simulink model "Model"  (R2021a)
settings: Solver=VariableStepAuto  StartTime=0.0  StopTime=1  RelTol=1e-3
PreLoadFcn:
  | Pmin = 50e3*.15;
  | V = 380;
  | f = 60;
  | fsw = 5e3;
  | Lf = ((.1*V^2)/(2*pi*f*Pmin));
  | RLf = Lf*25;
undefined symbols (not defined in the file or in its folder): sigbuilder_block
libraries: spsThreePhaseSeriesRLCLoadLib x11, spsThreePhaseVIMeasurementLib x4, spsThreePhaseHarmonicFilterLib x3, spsIdealSwitchLib x3, pid_lib x2, spsThreePhaseBreakerLib x1, spsImpedanceMeasurementLib x1, spsPWMGenerator2LevelLib x1, spsThreePhaseSeriesRLCBranchLib x1, spsUniversalBridgeLib x1, spsabctodq0Lib x1, spsdq0toabcLib x1
settings Model: Creator=SHANTO  LastModifiedBy=SHANTO

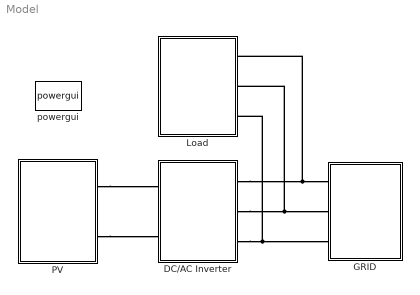
== system Model ==
  DC/AC Inverter : Subsystem
      mask Display: image('$imagefile'); % Use "Edit Image" on toolstrip to change.
  GRID : Subsystem
      mask Display: image('$imagefile'); % Use "Edit Image" on toolstrip to change.
  Load : Subsystem
      mask Display: image('$imagefile'); % Use "Edit Image" on toolstrip to change.
  "PV " : Subsystem
      mask Display: image('$imagefile'); % Use "Edit Image" on toolstrip to change.
  powergui : spspowerguiLib/powergui  Priority=1  SimulationMode=Discrete  SampleTime=1e-06  frequency=60  Iterations=50  frequencyindice=0  Pbase=100e6  ErrMax=1e-4  UnitsV=kV  UnitsW=MW  buscounter=0  FunctionMessages=off  echomessages=off  EnableUseOfTLC=off  CurrentSourceSwitches=off  DisableSnubberDevices=off  DisableRonSwitches=off  DisableVfSwitches=off  DisplayEquations=off  AutomaticDiscreteSolvers=off  SolverType=Tustin/Backward Euler (TBE)  Interpol=off  ExternalGateDelay=off  methode=off  Ts=100  x0status=blocks  SPID=on  SwTol=0  HookPort=off  NonlinearTolerance=1e-4  nMaxIteration=100  ContinueOnMaxIteration=off  RestoreLinks=warning  ResistiveCurrentMeasurement=off  Frange=[0:2:500]  Ylog=off  Xlog=on  ShowGrid=off  save=off  variable=ZData  structure=0  ZoomFFT=off  StartTime=0.0  cycles=1  DisplayStyle=1  fundamental=60  FreqAxis=off  MaxFrequency=1000  frequencyindicesteady=1  RmsSteady=1  display=off
  connections:
  "PV "/RConn1 -- DC/AC Inverter/LConn1
  "PV "/RConn2 -- DC/AC Inverter/LConn2
  DC/AC Inverter/RConn1 -- Load/RConn1 -- GRID/LConn1
  DC/AC Inverter/RConn2 -- GRID/LConn2 -- Load/RConn2
  DC/AC Inverter/RConn3 -- GRID/LConn3 -- Load/RConn3

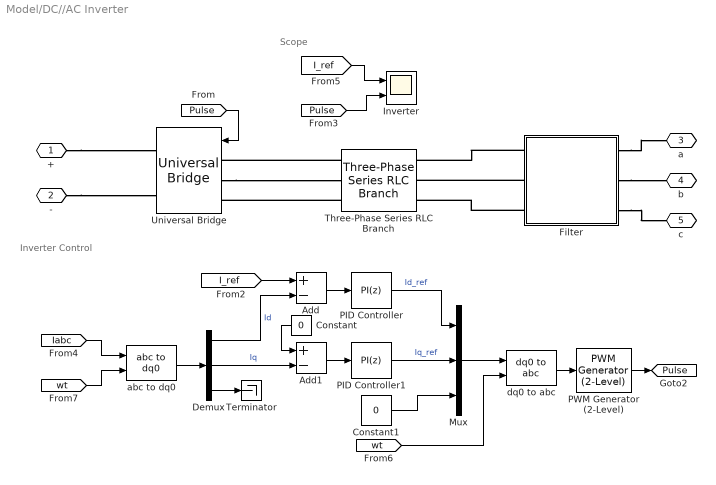
== system Model/DC//AC Inverter ==
  note: Scope
  note: Inverter Control
  Add : Sum  Inputs=+-
  Add1 : Sum  Inputs=+-
  Constant : Constant  Value=0
  Constant1 : Constant  Value=0
  Demux : Demux  Outputs=3
  Filter : Subsystem
  Inverter : Scope  NumInputPorts=2
  Mux : Mux  Inputs=3
  PID Controller : pid_lib/PID Controller  Controller=PI  Form=Parallel  TimeDomain=Discrete-time  UseExternalTs=off  SampleTime=1e-06  IntegratorMethod=Forward Euler  FilterMethod=Forward Euler  ControllerParametersSource=internal  P=0.005  I=1  D=0  UseFilter=on  N=100  TunerSelectOption=Transfer Function Based (PID Tuner App)  InitialConditionSource=internal  InitialConditionForIntegrator=0  InitialConditionForFilter=0  DifferentiatorICPrevScaledInput=0  ExternalReset=none  TrackingMode=off  Kt=1  LimitOutput=on  SatLimitsSource=internal  UpperSaturationLimit=1.2  LowerSaturationLimit=0  LinearizeAsGain=on  AntiWindupMode=none  Kb=1  POutMin=[]  POutMax=[]  IOutMin=[]  IOutMax=[]  DOutMin=[]  DOutMax=[]  NOutMin=[]  NOutMax=[]  SumOutMin=[]  SumOutMax=[]  SaturationOutMin=[]  SaturationOutMax=[]  PParamMin=[]  PParamMax=[]  IParamMin=[]  IParamMax=[]  DParamMin=[]  DParamMax=[]  NParamMin=[]  NParamMax=[]  KbParamMin=[]  KbParamMax=[]  KtParamMin=[]  KtParamMax=[]  KbOutMin=[]  KbOutMax=[]  KtOutMin=[]  KtOutMax=[]  IntegratorOutMin=[]  IntegratorOutMax=[]  FilterOutMin=[]  FilterOutMax=[]  SumI1OutMin=[]  SumI1OutMax=[]  SumI2OutMin=[]  SumI2OutMax=[]  SumI3OutMin=[]  SumI3OutMax=[]  SumI4OutMin=[]  SumI4OutMax=[]  SumDOutMin=[]  SumDOutMax=[]  DifferentiatorOutMin=[]  DifferentiatorOutMax=[]  FilterDiffOutCoefMin=[]  FilterDiffOutCoefMax=[]  ReciprocalOutMin=[]  ReciprocalOutMax=[]  SumDenOutMin=[]  SumDenOutMax=[]  SumNumOutMin=[]  SumNumOutMax=[]  DivideOutMin=[]  DivideOutMax=[]  UdiffTsProdOutMin=[]  UdiffTsProdOutMax=[]  NTsProdOutMin=[]  NTsProdOutMax=[]  UintegralTsProdOutMin=[]  UintegralTsProdOutMax=[]  UngainTsProdOutMin=[]  UngainTsProdOutMax=[]  IntegratorContinuousStateAttributes=''  IntegratorStateMustResolveToSignalObject=off  IntegratorRTWStateStorageClass=Auto  FilterContinuousStateAttributes=''  FilterStateMustResolveToSignalObject=off  FilterRTWStateStorageClass=Auto  ParallelPVariant=InternalParameters  IdealPVariant=Disabled  IVariant=InternalParameters  DVariant=Disabled  IntegratorVariant=Discrete  SatVariant=Enabled  AWVariant=Passthrough  PCopyVariant=Disabled  TRVariant=Disabled  FdbkBlocksVariant=Forward  IdealPFdbkVariant=Disabled  SatFdbkVariant=Disabled  DerivativeFilterVariant=Disabled  NVariant=Disabled  NCopyVariant=Disabled_SignalSpec  FilterICVariant=Disabled  IntegratorICVariant=InternalICs  ExternalResetVariant=Disabled  TRSumVariant=Passthrough  SumFdbkVariant=Disabled  SumVariant=Sum_PI  TsampFilterVariant=InternalTs  TsampNgainVariant=Passthrough  TsampIntegralVariant=Passthrough  ExternalSaturationOutDataTypeStr=Inherit: Same as second input
  PID Controller1 : pid_lib/PID Controller  Controller=PI  Form=Parallel  TimeDomain=Discrete-time  UseExternalTs=off  SampleTime=1e-05  IntegratorMethod=Forward Euler  FilterMethod=Forward Euler  ControllerParametersSource=internal  P=0.005  I=1  D=0  UseFilter=on  N=100  TunerSelectOption=Transfer Function Based (PID Tuner App)  InitialConditionSource=internal  InitialConditionForIntegrator=0  InitialConditionForFilter=0  DifferentiatorICPrevScaledInput=0  ExternalReset=none  TrackingMode=off  Kt=1  LimitOutput=on  SatLimitsSource=internal  UpperSaturationLimit=1.2  LowerSaturationLimit=0  LinearizeAsGain=on  AntiWindupMode=none  Kb=1  POutMin=[]  POutMax=[]  IOutMin=[]  IOutMax=[]  DOutMin=[]  DOutMax=[]  NOutMin=[]  NOutMax=[]  SumOutMin=[]  SumOutMax=[]  SaturationOutMin=[]  SaturationOutMax=[]  PParamMin=[]  PParamMax=[]  IParamMin=[]  IParamMax=[]  DParamMin=[]  DParamMax=[]  NParamMin=[]  NParamMax=[]  KbParamMin=[]  KbParamMax=[]  KtParamMin=[]  KtParamMax=[]  KbOutMin=[]  KbOutMax=[]  KtOutMin=[]  KtOutMax=[]  IntegratorOutMin=[]  IntegratorOutMax=[]  FilterOutMin=[]  FilterOutMax=[]  SumI1OutMin=[]  SumI1OutMax=[]  SumI2OutMin=[]  SumI2OutMax=[]  SumI3OutMin=[]  SumI3OutMax=[]  SumI4OutMin=[]  SumI4OutMax=[]  SumDOutMin=[]  SumDOutMax=[]  DifferentiatorOutMin=[]  DifferentiatorOutMax=[]  FilterDiffOutCoefMin=[]  FilterDiffOutCoefMax=[]  ReciprocalOutMin=[]  ReciprocalOutMax=[]  SumDenOutMin=[]  SumDenOutMax=[]  SumNumOutMin=[]  SumNumOutMax=[]  DivideOutMin=[]  DivideOutMax=[]  UdiffTsProdOutMin=[]  UdiffTsProdOutMax=[]  NTsProdOutMin=[]  NTsProdOutMax=[]  UintegralTsProdOutMin=[]  UintegralTsProdOutMax=[]  UngainTsProdOutMin=[]  UngainTsProdOutMax=[]  IntegratorContinuousStateAttributes=''  IntegratorStateMustResolveToSignalObject=off  IntegratorRTWStateStorageClass=Auto  FilterContinuousStateAttributes=''  FilterStateMustResolveToSignalObject=off  FilterRTWStateStorageClass=Auto  ParallelPVariant=InternalParameters  IdealPVariant=Disabled  IVariant=InternalParameters  DVariant=Disabled  IntegratorVariant=Discrete  SatVariant=Enabled  AWVariant=Passthrough  PCopyVariant=Disabled  TRVariant=Disabled  FdbkBlocksVariant=Forward  IdealPFdbkVariant=Disabled  SatFdbkVariant=Disabled  DerivativeFilterVariant=Disabled  NVariant=Disabled  NCopyVariant=Disabled_SignalSpec  FilterICVariant=Disabled  IntegratorICVariant=InternalICs  ExternalResetVariant=Disabled  TRSumVariant=Passthrough  SumFdbkVariant=Disabled  SumVariant=Sum_PI  TsampFilterVariant=InternalTs  TsampNgainVariant=Passthrough  TsampIntegralVariant=Passthrough  ExternalSaturationOutDataTypeStr=Inherit: Same as second input
  PWM Generator (2-Level) : spsPWMGenerator2LevelLib/PWM Generator (2-Level)  ModulatorType=Three-phase bridge (6 pulses)  ModulatorMode=Unsynchronized  Fc=fsw  Pc=90  nF=27  MinMax="[ -1  1 ]"  SamplingTechnique=Natural  ModulatingSignals=off  m=0.8  Freq=60  Phase=0  Ts=1e-6  ShowCarrierOutport=off
  Terminator : Terminator
  Three-Phase Series RLC Branch : spsThreePhaseSeriesRLCBranchLib/Three-Phase Series RLC Branch  LConnTagsString=A|B|C  RConnTagsString=A|B|C  BranchType=RL  Resistance=RLf  Inductance=Lf  Capacitance=1e-6  Measurements=None
  Universal Bridge : spsUniversalBridgeLib/Universal Bridge  Arms=3  SnubberResistance=1e5  SnubberCapacitance=inf  Device=IGBT / Diodes  Ron=1e-3  Lon=0  ForwardVoltages="[  0  0  ]"  ForwardVoltage=0  GTOparameters=[ 10e-6 , 20e-6 ]  IGBTparameters=[ 1e-6 , 2e-6 ]  Measurements=None  Measurements_2=None  converterType=Rectifier
  abc to dq0 : spsabctodq0Lib/abc to dq0  Alignment=90 degrees behind phase A axis
  dq0 to abc : spsdq0toabcLib/dq0 to abc  Alignment=90 degrees behind phase A axis
  + : PMIOPort  Side=Left
  - : PMIOPort  Port=2  Side=Left
  a : PMIOPort  Port=3  Side=Right
  b : PMIOPort  Port=4  Side=Right
  c : PMIOPort  Port=5  Side=Right
  tag scope: Pulse=global
  wires:
  [wt] -> abc to dq0/2
  Add1/1 -> PID Controller1/1
  Demux/2 -> Add1/2  "Iq"
  PID Controller1/1 -> Mux/2  "Iq_ref"
  PID Controller/1 -> Mux/1  "Id_ref"
  Constant/1 -> Add1/1
  Demux/1 -> Add/2  "Id"
  Add/1 -> PID Controller/1
  dq0 to abc/1 -> PWM Generator (2-Level)/1
  Mux/1 -> dq0 to abc/1
  Constant1/1 -> Mux/3
  abc to dq0/1 -> Demux/1
  [wt] -> dq0 to abc/2
  [Iabc] -> abc to dq0/1
  PWM Generator (2-Level)/1 -> [Pulse]
  Demux/3 -> Terminator/1
  [Pulse] -> Universal Bridge/1
  [I_ref] -> Add/1
  [I_ref] -> Inverter/1
  [Pulse] -> Inverter/2
  connections:
  Universal Bridge/LConn2 -- Three-Phase Series RLC Branch/LConn2
  Three-Phase Series RLC Branch/LConn3 -- Universal Bridge/LConn3
  -/RConn1 -- Universal Bridge/RConn2
  Filter/RConn2 -- Three-Phase Series RLC Branch/RConn2
  +/RConn1 -- Universal Bridge/RConn1
  Filter/RConn3 -- Three-Phase Series RLC Branch/RConn3
  Three-Phase Series RLC Branch/LConn1 -- Universal Bridge/LConn1
  Filter/RConn1 -- Three-Phase Series RLC Branch/RConn1
  Filter/LConn2 -- b/RConn1
  Filter/LConn1 -- a/RConn1
  Filter/LConn3 -- c/RConn1

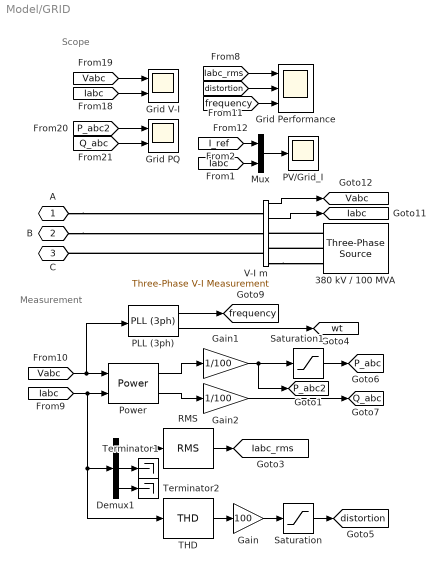
== system Model/GRID ==
  note: Scope
  note: Measurement
  380 kV / 100 MVA : spsThreePhaseSourceLib/Three-Phase Source  InternalConnection=Yg  VoltagePhases=off  Voltage=380  PhaseAngle=0  Voltage_phases=[25e3 25e3 25e3]/sqrt(3)  PhaseAngles_phases=[0 -120 +120]  Frequency=60  NonIdealSource=on  SpecifyImpedance=on  Resistance=1e-4  Inductance=0.2e-6  ShortCircuitLevel=100e6  BaseVoltage=380  XRratio=7  BusType=PQ  Pref=2.5e6  Qref=0  Prefabc=[10e3, 10e3, 10e3]  Qrefabc=[0, 0, 0]  Qmin=-inf  Qmax=inf
  Demux1 : Demux  Outputs=3
  Gain : Gain  Gain=100
  Gain1 : Gain  Gain=1/100
  Gain2 : Gain  Gain=1/100
  Grid PQ : Scope  NumInputPorts=2
  Grid Performance : Scope  NumInputPorts=3
  Grid V-I : Scope  NumInputPorts=2
  Mux : Mux  Inputs=2
  PLL (3ph) : spsPLL3phLib/PLL (3ph)  Fmin=45  Par_Init=[0, 60]  ParK=[180, 3200, 1]  TcD=1e-4  MaxRateChangeFreq=12  FilterCutOffFreq=25  Ts=1e-6  AGC=on
  PV/Grid_I : Scope
  Power : spsPowerLib/Power  Freq=60  Vinit=[1, 0]  Iinit=[1, 0]  Ts=0
      settings: SourceProductBaseCode=PS
  RMS : spsRMSLib/RMS  TrueRMS=on  Freq=60  RMSInit=120  Ts=1e-6
  Saturation : Saturate  UpperLimit=50  LowerLimit=0
  Saturation1 : Saturate  UpperLimit=60  LowerLimit=0
  THD : spsTHDLib/THD  Freq=60  Ts=1e-6
      settings: SourceProductBaseCode=PS
  Terminator1 : Terminator
  Terminator2 : Terminator
  V-I m : spsThreePhaseVIMeasurementLib/Three-Phase V-I Measurement  VoltageMeasurement=phase-to-ground  SetLabelV=off  LabelV=PV_Vabc  Vpu=off  VpuLL=off  CurrentMeasurement=yes  SetLabelI=off  LabelI=PV_Iabc  Ipu=off  Pbase=100e6  Vbase=500e3  OutputType=Complex  PhasorSimulation=off  PSBequivalent=0
  A : PMIOPort  Side=Left
  B : PMIOPort  Port=2  Side=Left
  C : PMIOPort  Port=3  Side=Left
  tag scope: Iabc=global, Iabc_rms=global, P_abc2=global, P_abc=global, Q_abc=global, Vabc=global, distortion=global, frequency=global, wt=global
  wires:
  V-I m/2 -> [Iabc]
  V-I m/1 -> [Vabc]
  [frequency] -> Grid Performance/3
  PLL (3ph)/2 -> [wt]
  PLL (3ph)/1 -> [frequency]
  [distortion] -> Grid Performance/2
  Power/2 -> Gain2/1
  Gain2/1 -> [Q_abc]
  [Iabc_rms] -> Grid Performance/1
  Demux1/1 -> RMS/1
  Power/1 -> Gain1/1
  THD/1 -> Gain/1
  Demux1/2 -> Terminator1/1
  [Iabc] -> Power/2, THD/1, Demux1/1
  [Vabc] -> PLL (3ph)/1, Power/1
  Demux1/3 -> Terminator2/1
  Saturation1/1 -> [P_abc]
  Gain/1 -> Saturation/1
  Gain1/1 -> [P_abc2], Saturation1/1
  Saturation/1 -> [distortion]
  RMS/1 -> [Iabc_rms]
  [Vabc] -> Grid V-I/1
  [Iabc] -> Grid V-I/2
  [Q_abc] -> Grid PQ/2
  [P_abc2] -> Grid PQ/1
  Mux/1 -> PV/Grid_I/1
  [Iabc] -> Mux/2
  [I_ref] -> Mux/1
  connections:
  380 kV / 100 MVA/RConn1 -- V-I m/RConn1
  V-I m/RConn3 -- 380 kV / 100 MVA/RConn3
  380 kV / 100 MVA/RConn2 -- V-I m/RConn2
  A/RConn1 -- V-I m/LConn1
  B/RConn1 -- V-I m/LConn2
  V-I m/LConn3 -- C/RConn1

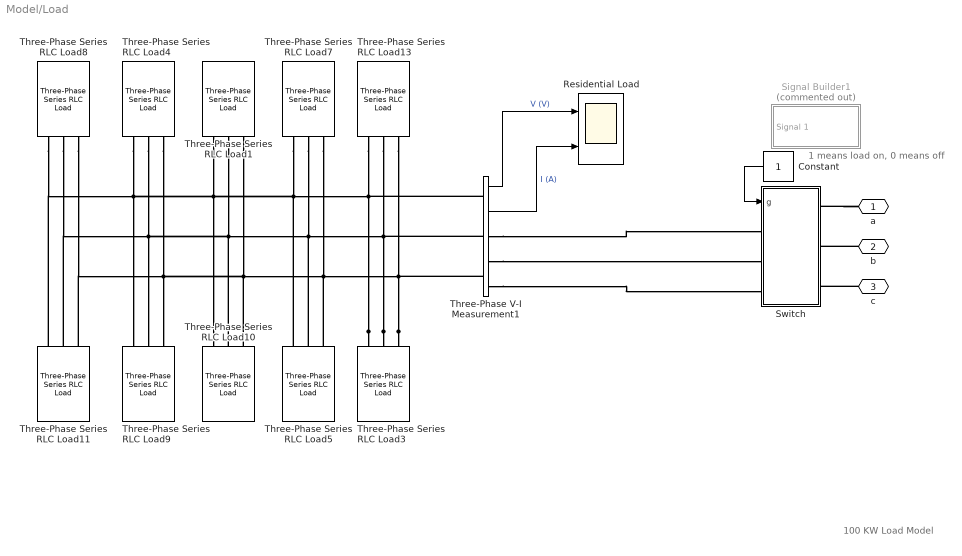
== system Model/Load ==
  note: 1 means load on, 0 means off
  note: 100 KW Load Model
  Constant : Constant
  Residential Load : Scope  NumInputPorts=2
  Signal Builder1 : Subsystem  Tag=STV Subsys  Commented=on  LoadFcn=sigbuilder_block('load');  StartFcn=sigbuilder_block('start');  StopFcn=sigbuilder_block('stop');  ClipboardFcn=sigbuilder_block('clipboard');  mask(Sigbuilder block){tuvar=[0:10]}
      mask help: Simulink:masks:SigbuilderBlock_MD
      mask init:
      | if ~strcmp(get_param(bdroot(gcbh),'SimulationStatus'),'stopped') tuvar = sigbuilder_block('maskInit'); end
      settings: CopyFcn=sigbuilder_block('copy');  DeleteFcn=sigbuilder_block('delete');  ModelCloseFcn=sigbuilder_block('modelClose');  PreSaveFcn=sigbuilder_block('preSave');  PauseFcn=sigbuilder_block('pause');  ContinueFcn=sigbuilder_block('continue');  NameChangeFcn=sigbuilder_block('namechange');  OpenFcn=sigbuilder_block('open',[437.6 199.2 550.4 400 ]);  CloseFcn=sigbuilder_block('close');
      mask Display: plot(0, 0, 100, 100,[2, 2, 32, 32, 2], [68, 8, 8, 68, 68],[32, 2], [38, 38], [32, 19, 2],[53, 60, 44], [32, 17, 17, 2],[16, 16, 31, 31]);txt = getActiveGroup(gcbh);text(2, 100, txt,'verticalAlignment', 'top');
  Switch : Subsystem
  Three-Phase Series RLC Load{1,3..5,7..11,13} (10 alike) : spsThreePhaseSeriesRLCLoadLib/Three-Phase Series RLC Load  LConnTagsString=A|B|C  Configuration=Y (grounded)  NominalVoltage=380  Vabc=[1e3 1e3 1e3]  Vabcp=[1e3 1e3 1e3]  NominalFrequency=60  UnbalancedPower=off  ActivePower=10e3  InductivePower=100  CapacitivePower=100  Pabc=[10e3 9e3 11e3]  QLabc=[100 90 110]  QCabc=[100 90 110]  Pabcp=[10e3 9e3 11e3]  QLabcp=[100 90 110]  QCabcp=[100 90 110]  Measurements=None  LoadType=constant Z
  Three-Phase V-I Measurement1 : spsThreePhaseVIMeasurementLib/Three-Phase V-I Measurement  VoltageMeasurement=phase-to-ground  SetLabelV=off  LabelV=Vabc_load2  Vpu=off  VpuLL=off  CurrentMeasurement=yes  SetLabelI=off  LabelI=Iabc_load2  Ipu=off  Pbase=100e6  Vbase=500e3  OutputType=Complex  PhasorSimulation=off  PSBequivalent=0
  a : PMIOPort  Side=Right
  b : PMIOPort  Port=2  Side=Right
  c : PMIOPort  Port=3  Side=Right
  wires:
  Three-Phase V-I Measurement1/2 -> Residential Load/2  "I (A)"
  Three-Phase V-I Measurement1/1 -> Residential Load/1  "V (V)"
  Constant/1 -> Switch/1(g)
  connections:
  Three-Phase V-I Measurement1/RConn3 -- Switch/LConn3
  Three-Phase Series RLC Load3/LConn1 -- Three-Phase V-I Measurement1/LConn1 -- Three-Phase Series RLC Load13/LConn1 -- Three-Phase Series RLC Load8/LConn1 -- Three-Phase Series RLC Load11/LConn1 -- Three-Phase Series RLC Load4/LConn1 -- Three-Phase Series RLC Load9/LConn1 -- Three-Phase Series RLC Load1/LConn1 -- Three-Phase Series RLC Load10/LConn1 -- Three-Phase Series RLC Load7/LConn1 -- Three-Phase Series RLC Load5/LConn1
  Three-Phase V-I Measurement1/RConn2 -- Switch/LConn2
  Three-Phase Series RLC Load3/LConn3 -- Three-Phase Series RLC Load10/LConn3 -- Three-Phase Series RLC Load8/LConn3 -- Three-Phase Series RLC Load11/LConn3 -- Three-Phase Series RLC Load4/LConn3 -- Three-Phase Series RLC Load9/LConn3 -- Three-Phase Series RLC Load1/LConn3 -- Three-Phase Series RLC Load7/LConn3 -- Three-Phase Series RLC Load5/LConn3 -- Three-Phase V-I Measurement1/LConn3 -- Three-Phase Series RLC Load13/LConn3
  Three-Phase Series RLC Load3/LConn2 -- Three-Phase V-I Measurement1/LConn2 -- Three-Phase Series RLC Load13/LConn2 -- Three-Phase Series RLC Load8/LConn2 -- Three-Phase Series RLC Load11/LConn2 -- Three-Phase Series RLC Load4/LConn2 -- Three-Phase Series RLC Load9/LConn2 -- Three-Phase Series RLC Load1/LConn2 -- Three-Phase Series RLC Load10/LConn2 -- Three-Phase Series RLC Load7/LConn2 -- Three-Phase Series RLC Load5/LConn2
  Three-Phase V-I Measurement1/RConn1 -- Switch/LConn1
  c/RConn1 -- Switch/RConn3
  b/RConn1 -- Switch/RConn2
  a/RConn1 -- Switch/RConn1

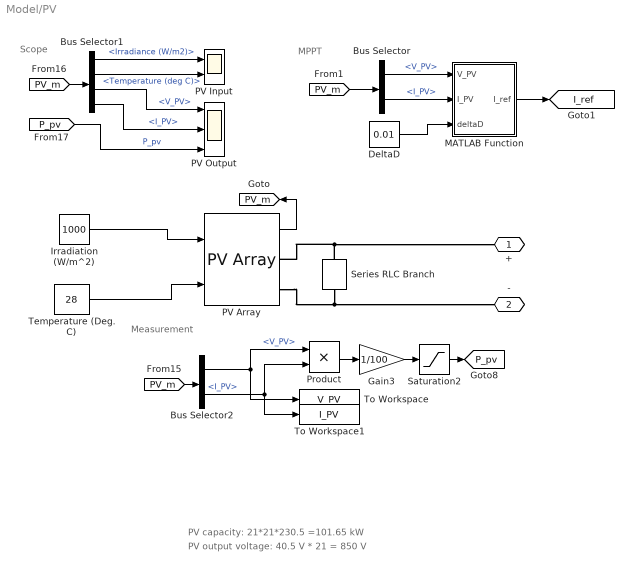
== system Model/PV  ==
  note: PV output voltage: 40.5 V * 21 = 850 V
  note: PV capacity: 21*21*230.5 =101.65 kW
  note: Scope
  note: Measurement
  note: MPPT
  Bus Selector : BusSelector  OutputSignals=V_PV,I_PV
  Bus Selector1 : BusSelector  OutputSignals=Irradiance (W/m2),Temperature (deg C),V_PV,I_PV
  Bus Selector2 : BusSelector  OutputSignals=V_PV,I_PV
  DeltaD : Constant  Value=0.01
  Gain3 : Gain  Gain=1/100
  Irradiation (W/m^2) : Constant  Value=1000
  MATLAB Function : MATLAB Function  TreatAsAtomicUnit=on
  PV Array : spsPVArrayLib/PV Array  Npar=21  Nser=21  PlotType=one module @ 25 deg.C & specified irradiances  S_vec=[1000 600 400 100]  Temp_C_vec="[ 45 25  ]"  ModuleName=SunPower SPR-230E-WHT-D  PlotWhenSelected=off  Pm=230.04  Ncell=72  Voc=48.2  Isc=6.05  Vm=40.5  Im=5.68  beta_Voc_pc=-0.31  alpha_Isc_pc=0.016  beta_Voc=-0.14942  alpha_Isc=0.000968  IL=6.0553  I0=2.9343e-11  nI=1.0009  Rsh=396.8073  Rs=0.34627  RobustModel=off  RobustCellTemperature=313.3991  BAL=on  Tc=1e-6  Tfilter=5e-5
  PV Input : Scope  NumInputPorts=2
  PV Output : Scope  NumInputPorts=3
  Product : Product
  Saturation2 : Saturate  UpperLimit=60  LowerLimit=0
  Series RLC Branch : spsSeriesRLCBranchLib/Series RLC Branch  LConnTagsString=__new0  RConnTagsString=__new0  BranchType=RC  Resistance=1e-3  Inductance=1e-3  SetiL0=off  InitialCurrent=0  Capacitance=100e-6  Setx0=off  InitialVoltage=0  Measurements=None
  Temperature (Deg. C) : Constant  Value=28
  To Workspace : ToWorkspace  VariableName=V_PV  SaveFormat=Timeseries  SampleTime=-1
  To Workspace1 : ToWorkspace  VariableName=I_PV  SaveFormat=Timeseries  SampleTime=-1
  + : PMIOPort  Side=Right
  - : PMIOPort  Port=2  Side=Right
  tag scope: I_ref=global, PV_m=global, P_pv=global
  wires:
  PV Array/1 -> [PV_m]
  [P_pv] -> PV Output/3  "P_pv"
  [PV_m] -> Bus Selector1/1
  Irradiation (W/m^2)/1 -> PV Array/1
  Temperature (Deg. C)/1 -> PV Array/2
  Saturation2/1 -> [P_pv]
  Gain3/1 -> Saturation2/1
  [PV_m] -> Bus Selector2/1
  Bus Selector2/1 -> Product/1, To Workspace/1  "<V_PV>"
  Bus Selector2/2 -> Product/2, To Workspace1/1  "<I_PV>"
  Product/1 -> Gain3/1
  Bus Selector/2 -> MATLAB Function/2(I_PV)  "<I_PV>"
  Bus Selector/1 -> MATLAB Function/1(V_PV)  "<V_PV>"
  [PV_m] -> Bus Selector/1
  DeltaD/1 -> MATLAB Function/3(deltaD)
  MATLAB Function/1(I_ref) -> [I_ref]
  Bus Selector1/1 -> PV Input/1  "<Irradiance (W/m2)>"
  Bus Selector1/2 -> PV Input/2  "<Temperature (deg C)>"
  Bus Selector1/3 -> PV Output/1  "<V_PV>"
  Bus Selector1/4 -> PV Output/2  "<I_PV>"
  connections:
  Series RLC Branch/RConn1 -- PV Array/RConn2 -- -/RConn1
  Series RLC Branch/LConn1 -- +/RConn1 -- PV Array/RConn1

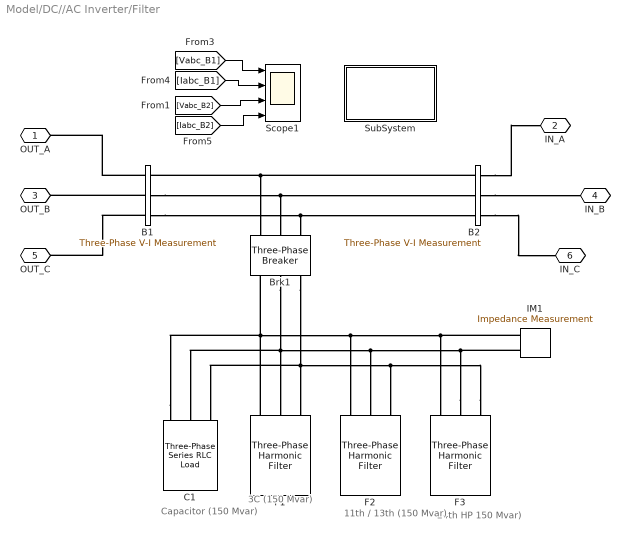
== system Model/DC//AC Inverter/Filter ==
  note: Capacitor
      | (150 Mvar)
  note: 24th HP
      | 150 Mvar)
  note: 11th / 13th
      | (150 Mvar)
  note: 3C
      | (150 Mvar)
  B1 : spsThreePhaseVIMeasurementLib/Three-Phase V-I Measurement  VoltageMeasurement=phase-to-ground  SetLabelV=on  LabelV=Vabc_B1  Vpu=off  VpuLL=off  CurrentMeasurement=yes  SetLabelI=on  LabelI=Iabc_B1  Ipu=off  Pbase=100e6  Vbase=500e3  OutputType=Magnitude  PhasorSimulation=off  PSBequivalent=0
  "B2 " : spsThreePhaseVIMeasurementLib/Three-Phase V-I Measurement  VoltageMeasurement=phase-to-ground  SetLabelV=on  LabelV=Vabc_B2  Vpu=off  VpuLL=off  CurrentMeasurement=yes  SetLabelI=on  LabelI=Iabc_B2  Ipu=off  Pbase=100e6  Vbase=500e3  OutputType=Magnitude  PhasorSimulation=off  PSBequivalent=0
  Brk1 : spsThreePhaseBreakerLib/Three-Phase Breaker  InitialState=closed  SwitchA=off  SwitchB=off  SwitchC=off  SwitchTimes="[4/60  10/60]"  External=off  BreakerResistance=1e-4  SnubberResistance=1e6  SnubberCapacitance=inf  Measurements=None
      settings: AttributesFormatString=\n
  C1 : spsThreePhaseSeriesRLCLoadLib/Three-Phase Series RLC Load  LConnTagsString=A|B|C  Configuration=Y (grounded)  NominalVoltage=500e3  Vabc=[1e3 1e3 1e3]  Vabcp=[1e3 1e3 1e3]  NominalFrequency=60  UnbalancedPower=off  ActivePower=0  InductivePower=0  CapacitivePower=150e6  Pabc=[10e3 9e3 11e3]  QLabc=[100 90 110]  QCabc=[100 90 110]  Pabcp=[10e3 9e3 11e3]  QLabcp=[100 90 110]  QCabcp=[100 90 110]  Measurements=None  LoadType=constant Z
  "F1 " : spsThreePhaseHarmonicFilterLib/Three-Phase Harmonic Filter  LConnTagsString=A|B|C  FilterType=C-type High-pass  FilterConnection=Y (grounded)  ParNom=[500e3 60]  Qc=150e6  Fr=[3*60]  Frd=[11*60 13*60]  Q=2  Measurements=None
      settings: AttributesFormatString=\n  SourceProductBaseCode=PS
  F2 : spsThreePhaseHarmonicFilterLib/Three-Phase Harmonic Filter  LConnTagsString=A|B|C  FilterType=Double-tuned  FilterConnection=Y (grounded)  ParNom=[500e3 60]  Qc=150e6  Fr=[3*60]  Frd=[11*60 13*60]  Q=20  Measurements=None
      settings: AttributesFormatString=\n  SourceProductBaseCode=PS
  F3 : spsThreePhaseHarmonicFilterLib/Three-Phase Harmonic Filter  LConnTagsString=A|B|C  FilterType=High-pass  FilterConnection=Y (grounded)  ParNom=[500e3 60]  Qc=150e6  Fr=[24*60]  Frd=[11*60 13*60]  Q=7  Measurements=None
      settings: AttributesFormatString=\n  SourceProductBaseCode=PS
  IM1 : spsImpedanceMeasurementLib/Impedance Measurement  LConnTagsString=+|-  Factor=0.5
      settings: SourceProductBaseCode=PS
  Scope1 : Scope  NumInputPorts=4
  SubSystem : Subsystem
      settings: OpenFcn=openfig('filters_impedance.fig');
      mask Display: disp('Show\nfilters impedance\nvs\nfrequency')
  OUT_A : PMIOPort  Side=Left
  IN_A : PMIOPort  Port=2  Side=Right
  OUT_B : PMIOPort  Port=3  Side=Left
  IN_B : PMIOPort  Port=4  Side=Right
  OUT_C : PMIOPort  Port=5  Side=Left
  IN_C : PMIOPort  Port=6  Side=Right
  wires:
  [Vabc_B1] -> Scope1/1
  [Iabc_B1] -> Scope1/2
  [Vabc_B2] -> Scope1/3
  [Iabc_B2] -> Scope1/4
  connections:
  B1/RConn2 -- Brk1/LConn2 -- "B2 "/LConn2
  "B2 "/LConn1 -- Brk1/LConn1 -- B1/RConn1
  F3/LConn2 -- IM1/LConn2 -- F2/LConn2 -- Brk1/RConn2 -- C1/LConn2 -- "F1 "/LConn2
  C1/LConn1 -- "F1 "/LConn1 -- F2/LConn1 -- IM1/LConn1 -- F3/LConn1 -- Brk1/RConn1
  F3/LConn3 -- F2/LConn3 -- Brk1/RConn3 -- C1/LConn3 -- "F1 "/LConn3
  B1/RConn3 -- Brk1/LConn3 -- "B2 "/LConn3
  "B2 "/RConn3 -- IN_C/RConn1
  B1/LConn1 -- OUT_A/RConn1
  "B2 "/RConn1 -- IN_A/RConn1
  "B2 "/RConn2 -- IN_B/RConn1
  B1/LConn2 -- OUT_B/RConn1
  B1/LConn3 -- OUT_C/RConn1

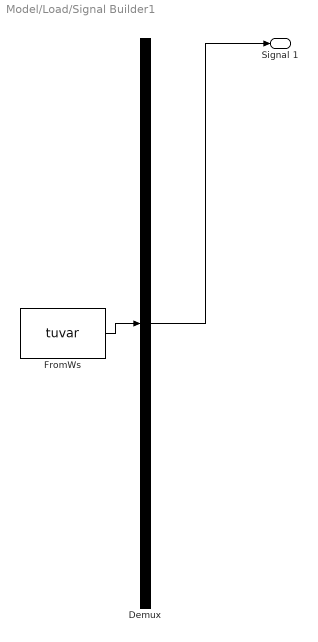
== system Model/Load/Signal Builder1 ==
  Demux : Demux  Tag=STV Demux  Outputs=1
      settings: DisplayOption=none
  FromWs : FromWorkspace  Tag=STV FromWs  VariableName=tuvar
      SigBuilderData=|
      | common.afterFinalStr = 'Extrapolate'
      | common.sampleTime = 0
      | dataSet.timeRange = [0 10]
      | dataSet.name = 'Group 1'
      | sbobj.Groups.Name = 'Group 1'
      | sbobj.Groups.Signals.Name = 'Signal 1'
      | sbobj.Groups.Signals.XData = [0 0.36 0.36 9.78 9.78 10]
      | sbobj.Groups.Signals.YData = [0 0 1 1 0 0]
  Signal 1 : Outport  Tag=STV Outport
  wires:
  Demux/1 -> Signal 1/1
  FromWs/1 -> Demux/1

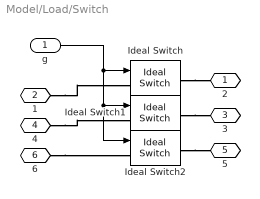
== system Model/Load/Switch ==
  g : Inport
  Ideal Switch : spsIdealSwitchLib/Ideal Switch  Ron=0.001  Lon=0  IC=0  Rs=1e5  Cs=inf  Measurements=off
  Ideal Switch1 : spsIdealSwitchLib/Ideal Switch  Ron=0.001  Lon=0  IC=0  Rs=1e5  Cs=inf  Measurements=off
  Ideal Switch2 : spsIdealSwitchLib/Ideal Switch  Ron=0.001  Lon=0  IC=0  Rs=1e5  Cs=inf  Measurements=off
  2 : PMIOPort  Side=Right
  1 : PMIOPort  Port=2  Side=Left
  3 : PMIOPort  Port=3  Side=Right
  4 : PMIOPort  Port=4  Side=Left
  5 : PMIOPort  Port=5  Side=Right
  6 : PMIOPort  Port=6  Side=Left
  wires:
  g/1 -> Ideal Switch2/1, Ideal Switch1/1, Ideal Switch/1
  connections:
  6/RConn1 -- Ideal Switch2/LConn1
  Ideal Switch2/RConn1 -- 5/RConn1
  1/RConn1 -- Ideal Switch/LConn1
  Ideal Switch/RConn1 -- 2/RConn1
  4/RConn1 -- Ideal Switch1/LConn1
  Ideal Switch1/RConn1 -- 3/RConn1

== system Model/DC//AC Inverter/Filter/SubSystem ==

== matlab function Model/PV /MATLAB Function ==
  data: V_PV input; I_ref output; I_PV input; deltaD input
function I_ref = mppt_alg(V_PV, I_PV, deltaD)

Iref_init = 100;
I_min = 0;
I_max = 150;

persistent Vold Pold Iref_old;

% dataType = 'double';

if isempty(Vold)
    Vold = 0;
    Pold = 0;
    Iref_old = Iref_init;
end

P = V_PV*I_PV;
dV = V_PV-Vold;
dP = P-Pold;
I_ref = Iref_old;

if dP ~= 0 && V_PV > 400
    if dP < 0
        if dV < 0
            I_ref = Iref_old - deltaD;
        else
            I_ref = Iref_old + deltaD;
        end
    else 
        if dV < 0
            I_ref = Iref_old + deltaD;
        else
            I_ref = Iref_old - deltaD;
        end
    end
end

if I_ref >= I_max  
    I_ref = I_max;
end

if I_ref < I_min 
    I_ref = I_min;
end

Iref_old = I_ref;
Vold = V_PV;
Pold = P;
end
